simulink model "slb_add_mult"  (R2015b)
settings: Solver=FixedStepDiscrete  SolverMode=SingleTasking  StartTime=0.0  StopTime=3  RelTol=1e-3
settings Model: Creator=at-mt  LastModifiedBy=amatsumo
settings DataIOCC: SaveFormat=Array  SignalLoggingSaveFormat=ModelDataLogs  SaveOutput=off  SignalLogging=off  SaveTime=off
settings OptimizationCC: BlockReduction=off  ConditionallyExecuteInputs=off  DefaultParameterBehavior=Inlined  ExpressionDepthLimit=2147483647
settings DebuggingCC: AlgebraicLoopMsg=error  UnderspecifiedInitializationDetection=Classic  MergeDetectMultiDrivingBlocksExec=none  SolverPrmCheckMsg=warning  SingleTaskRateTransMsg=error  FcnCallInpInsideContextMsg=UseLocalSettings  StateNameClashWarn=warning
settings HardwareCC: ProdBitPerPointer=32  ProdLargestAtomicFloat=None  ProdIntDivRoundTo=Undefined  ProdEndianess=Unspecified  ProdWordSize=32  ProdHWDeviceType=ASIC/FPGA->ASIC/FPGA  ProdEqTarget=off
settings SFSimCC: SFSimEcho=off
settings GRTTargetCC: GeneratePreprocessorConditionals=Disable all  CombineOutputUpdateFcns=off  GRTInterface=on
settings ConfigComp: CovModelRefEnable=Off  CovSFcnEnable=off

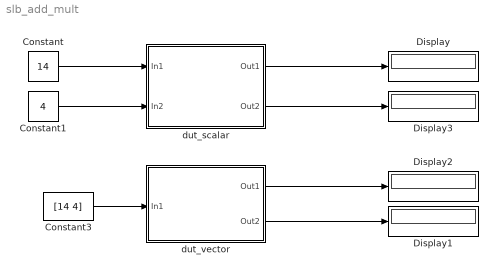
== system slb_add_mult ==
  Constant : Constant  Value=14  OutDataTypeStr=int8  SampleTime=1
  Constant1 : Constant  Value=4  OutDataTypeStr=int8  SampleTime=1
  Constant3 : Constant  Value=[14 4]  OutDataTypeStr=int8  SampleTime=1
  Display{,1..3} (4 alike) : Display
  dut_scalar : Subsystem
  dut_vector : Subsystem
  wires:
  Constant/1 -> dut_scalar/1(In1)
  Constant1/1 -> dut_scalar/2(In2)
  dut_scalar/1(Out1) -> Display/1
  Constant3/1 -> dut_vector/1(In1)
  dut_vector/2(Out2) -> Display1/1
  dut_vector/1(Out1) -> Display2/1
  dut_scalar/2(Out2) -> Display3/1

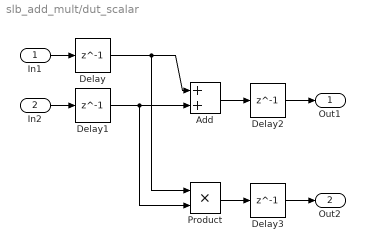
== system slb_add_mult/dut_scalar ==
  In1 : Inport
  In2 : Inport  Port=2
  Add : Sum
  Delay{,1..3} (4 alike) : Delay  DelayLength=1
  Product : Product  RndMeth=Zero
  Out1 : Outport
  Out2 : Outport  Port=2
  wires:
  Delay/1 -> Product/1, Add/1
  Delay1/1 -> Product/2, Add/2
  Product/1 -> Delay3/1
  In1/1 -> Delay/1
  In2/1 -> Delay1/1
  Add/1 -> Delay2/1
  Delay2/1 -> Out1/1
  Delay3/1 -> Out2/1

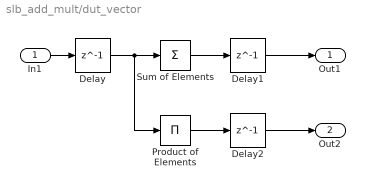
== system slb_add_mult/dut_vector ==
  In1 : Inport
  Delay : Delay  DelayLength=1
  Delay1 : Delay  DelayLength=1
  Delay2 : Delay  DelayLength=1
  Product of Elements : Product  Inputs=*
  Sum of Elements : Sum  Inputs=+
  Out1 : Outport
  Out2 : Outport  Port=2
  wires:
  In1/1 -> Delay/1
  Product of Elements/1 -> Delay2/1
  Sum of Elements/1 -> Delay1/1
  Delay/1 -> Product of Elements/1, Sum of Elements/1
  Delay1/1 -> Out1/1
  Delay2/1 -> Out2/1
